simulink model "LCD1602_int2string"  (R2016b)
settings: Solver=FixedStepAuto  StartTime=0.0  StopTime=inf  RelTol=1e-3  EnableMultiTasking=on
PreLoadFcn:
  | addpath(genpath('../../Drivers'))
libraries: arduinoDrivers_lib x5
settings Model: SimulationMode=external  ExtModeTrigDuration=2  Creator=Raphael  LastModifiedBy=Raphael
settings OptimizationCC: MaxStackSize=64
settings DebuggingCC: ParameterTunabilityLossMsg=error
settings HardwareCC: ProdBitPerInt=16  ProdBitPerPointer=16  ProdBitPerSizeT=16  ProdBitPerPtrDiffT=16  ProdLargestAtomicFloat=None  ProdWordSize=8  ProdHWDeviceType=Atmel->AVR
settings RTWCC: SystemTargetFile=ert.tlc  HardwareBoard=Arduino Mega 2560  TLCOptions=-aInlineSetEventsForThisBaseRateFcn=TLC_FALSE -aSuppressMultiTaskScheduler=TLC_FALSE -aRateBasedStepFcn=1  TemplateMakefile=ert_default_tmf  Description=Embedded Coder  GenerateReport=on  Toolchain=Arduino AVR v1.6.7  BuildConfiguration=Faster Runs  IncludeHyperlinkInReport=on  GenerateTraceInfo=on  GenerateTraceReport=on  GenerateTraceReportSl=on  GenerateTraceReportSf=on  GenerateTraceReportEml=on
settings CodeAppCC: ForceParamTrailComments=on  IgnoreCustomStorageClasses=off  OperatorAnnotations=on  SimulinkDataObjDesc=on  SFDataObjDesc=on  MATLABFcnDesc=on  InsertBlockDesc=on  MATLABSourceComments=on
settings ERTTargetCC: SupportContinuousTime=on  SupportVariableSizeSignals=on

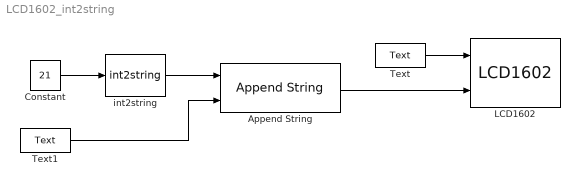
== system LCD1602_int2string ==
  Append String : arduinoDrivers_lib/LCD1602 16x2 LiquidCrystal-Display/Append String
  Constant : Constant  Value=21  OutDataTypeStr=int8  SampleTime=2
  LCD1602 : arduinoDrivers_lib/LCD1602 16x2 LiquidCrystal-Display/LCD1602  rs_Mask=2  en_Mask=3  d4_Mask=4  d5_Mask=5  d6_Mask=6  d7_Mask=7
  Text : arduinoDrivers_lib/LCD1602 16x2 LiquidCrystal-Display/Text  text_Mask='Temperature:'  SampleTime=2
  Text1 : arduinoDrivers_lib/LCD1602 16x2 LiquidCrystal-Display/Text  text_Mask=' deg Celsius'  SampleTime=2
  int2string : arduinoDrivers_lib/LCD1602 16x2 LiquidCrystal-Display/int2string
  wires:
  Text/1 -> LCD1602/1
  Append String/1 -> LCD1602/2
  int2string/1 -> Append String/1
  Constant/1 -> int2string/1
  Text1/1 -> Append String/2
